simulink model "OBSERVATEUR"  (R2013a)
settings: Solver=ode45  StartTime=0.0  StopTime=10.0  RelTol=1e-3
values from neighbouring files (symbols this model uses):
  f = 7.26e-3    (= 0.00726)    [parametres.m]
  J = 0.038    [parametres.m]
  K = 0.74    [parametres.m]
  K1 = Kh*l1    (= -0.265728636842)    [parametres.m]
  K2 = -Kh*l2    (= 0.739115169049)    [parametres.m]
  Kh = 10    [parametres.m]
  L = 8.87e-3    (= 0.00887)    [parametres.m]
  R = 0.28    [parametres.m]
settings Model: Creator=ciottopinton_gus  LastModifiedBy=ciottopinton_gus

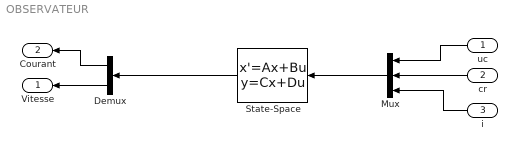
== system OBSERVATEUR ==
  uc : Inport
  cr : Inport  Port=2
  i : Inport  Port=3
  Demux : Demux  Outputs=2
  Mux : Mux  Inputs=3
  State-Space : StateSpace  A="[ [-(R + K1)/L  -K/L] ; [ (K - K2)/J -f/J ] ]"  B="[ [Kh/L 0 K1/L] ; [ 0 -1/J  K2/J ] ]"  C=[ 0 1 ]  D=[ 0 0 0 ]
  Vitesse : Outport
  Courant : Outport  Port=2
  wires:
  State-Space/1 -> Demux/1
  Mux/1 -> State-Space/1
  i/1 -> Mux/3
  cr/1 -> Mux/2
  uc/1 -> Mux/1
  Demux/2 -> Vitesse/1
  Demux/1 -> Courant/1
